simulink model "Fig34"  (R2022a)
settings: Solver=ode3  StartTime=0.0  StopTime=0.0150  FixedStep=2e-6  RelTol=1e-5  EnableMultiTasking=on
libraries: commfilt2 x1, commchan3 x1, commsink2 x1, commrandsrc2 x1
settings Model: Creator=Dennis Silage  LastModifiedBy=luanv
settings SolverCC: AlgebraicLoopSolver=TrustRegion
settings DataIOCC: LimitDataPoints=on  SaveFormat=Array  SignalLoggingSaveFormat=ModelDataLogs  ReturnWorkspaceOutputs=off
settings OptimizationCC: ExpressionDepthLimit=2147483647  InitFltsAndDblsToZero=on  LifeSpan=inf
settings DebuggingCC: UnderspecifiedInitializationDetection=Classic  MergeDetectMultiDrivingBlocksExec=none  FcnCallInpInsideContextMsg=warning  UnconnectedInputMsg=warning  UnconnectedOutputMsg=warning  UnconnectedLineMsg=warning  StateNameClashWarn=warning  SFUnexpectedBacktrackingDiag=warning  SFNoUnconditionalDefaultTransitionDiag=warning  SFExecutionAtInitializationDiag=none  SFMachineParentedDataDiag=warning  ArithmeticOperatorsInVariantConditions=warning
settings HardwareCC: ProdBitPerPointer=32  ProdBitPerSizeT=32  ProdBitPerPtrDiffT=32  ProdLargestAtomicFloat=None  ProdIntDivRoundTo=Undefined  ProdEndianess=Unspecified  ProdWordSize=32  ProdHWDeviceType=32-bit Generic
settings ModelReferenceCC: PropagateSignalLabelsOutOfModel=off
settings CodeAppCC: StateflowObjectComments=on
settings GRTTargetCC: TargetLangStandard=C89/C90 (ANSI)  CombineOutputUpdateFcns=off  GRTInterface=on
settings ConfigComp: CovMetricSettings=dw  CovSaveCumulativeToWorkspaceVar=on  CovSaveSingleToWorkspaceVar=on

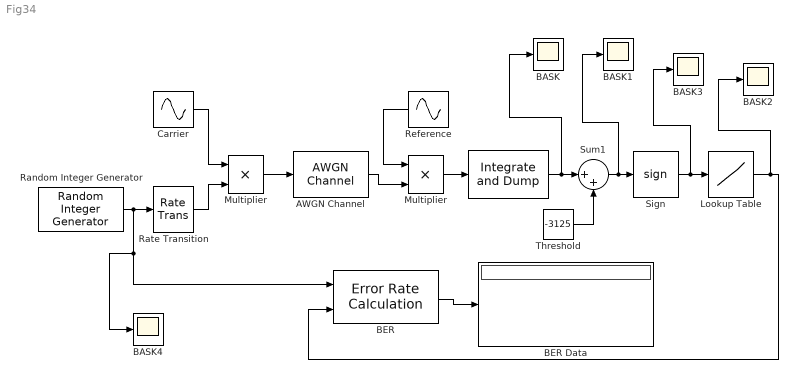
== system Fig34 ==
  " " : commfilt2/Integrate and Dump  obssamples=500  offsetsamples=0  nodump=off  roundingMode=Floor  overflowMode=off  outputDataTypeStr=Inherit: Same as accumulator  outputLastDataTypeStr=Inherit: Same as accumulator
  AWGN Channel : commchan3/AWGN Channel  InputProcessing=Columns as channels (frame based)  seed=153  noiseMode="Signal to noise ratio  (Eb/No)"  EbNodB=2  EsNodB=10  SNRdB=12  bitsPerSym=1  Ps=12.5  Tsym=1e-3  variance=0
  BASK{,1..4} (5 alike) : Scope
  BER : commsink2/Error Rate Calculation  N=2  st_delay=0  cp_mode=Entire frame  subframe=[]  PMode=Port  WsName=ErrorVec  RsMode2=off  stop=off  numErr=100  maxBits=1e6
  BER Data : Display
  Carrier : Sin  Amplitude=5  Frequency=40000*pi  SampleTime=2e-6
  Lookup Table : Lookup  InputValues=[-1,0,1]  Table=[0,0,1]  SaturateOnIntegerOverflow=off
  Multiplier : Product  RndMeth=Zero
  "Multiplier " : Product  RndMeth=Zero
  Random Integer Generator : commrandsrc2/Random Integer Generator  mul=2  seed=623642  Ts=1e-3  frameBased=off  sampPerFrame=50  orient=on  outDataType=double
      settings: SourceProductBaseCode=CM
  Rate Transition : RateTransition  OutPortSampleTime=2e-6
  Reference : Sin  Amplitude=5  Frequency=40000*pi  Samples=200  SampleTime=2e-6
  Sign : Signum
  Sum1 : Sum  Inputs=|++
  Threshold : Constant  Value=-3125
  wires:
  Sign/1 -> BASK3/1, Lookup Table/1
  Random Integer Generator/1 -> Rate Transition/1, BASK4/1, BER/1
  BER/1 -> BER Data/1
  Multiplier/1 -> " "/1
  AWGN Channel/1 -> Multiplier/2
  Threshold/1 -> Sum1/2
  Sum1/1 -> BASK1/1, Sign/1
  " "/1 -> BASK/1, Sum1/1
  "Multiplier "/1 -> AWGN Channel/1
  Reference/1 -> Multiplier/1
  Carrier/1 -> "Multiplier "/1
  Lookup Table/1 -> BASK2/1, BER/2
  Rate Transition/1 -> "Multiplier "/2
